simulink model "CM012A_FordT3McuCfg"  (R2013b)
settings: Solver=FixedStepDiscrete  SolverMode=SingleTasking  StartTime=0.0  StopTime=2  FixedStep=0.00005  RelTol=1e-3
values from neighbouring files (symbols this model uses):
  BATTVLTGSCAGFAC_ULS_F32 = DataDict.Constant    [CM012A_FordT3McuCfg_DataDict.m]
  BATTVLTGSWD1SCAGFAC_ULS_F32 = DataDict.Constant    [CM012A_FordT3McuCfg_DataDict.m]
  CHRGPMPDIAGSCAGFAC_ULS_F32 = DataDict.Constant    [CM012A_FordT3McuCfg_DataDict.m]
  MOTAG2MEAS_ECU1OFFS_MOTREV_F32 = DataDict.Constant    [CM012A_FordT3McuCfg_DataDict.m]
  MOTAG2MEAS_ECU2OFFS_MOTREV_F32 = DataDict.Constant    [CM012A_FordT3McuCfg_DataDict.m]
  PWRDISCNCTSWTDIAGSCAGFAC_ULS_F32 = DataDict.Constant    [CM012A_FordT3McuCfg_DataDict.m]
undefined symbols (not defined in the file or in its folder): HwAgSnsrTyp1, sigbuilder_block
libraries: CM012A_FordT3McuCfg_ModelLibrary x114, simulink x37, NxtrLim x34
(part 1 of 4)
settings Model: Creator=nz3zln  LastModifiedBy=NZ4630
settings SolverCC: AutoInsertRateTranBlk=on  InsertRTBMode=Always
settings DataIOCC: LimitDataPoints=off  SaveFormat=Structure  ReturnWorkspaceOutputs=on
settings OptimizationCC: BlockReduction=off  InlineParams=on  ZeroExternalMemoryAtStartup=off  ZeroInternalMemoryAtStartup=off  OptimizeModelRefInitCode=on  LifeSpan=1
settings DebuggingCC: SignalInfNanChecking=error  SignalRangeChecking=warning  UnderspecifiedInitializationDetection=Simplified  SolverPrmCheckMsg=error  InheritedTsInSrcMsg=error  DiscreteInheritContinuousMsg=error  MultiTaskRateTransMsg=warning  SingleTaskRateTransMsg=error  TasksWithSamePriorityMsg=error  SigSpecEnsureSampleTimeMsg=error  CheckMatrixSingularityMsg=error  ParameterUnderflowMsg=error  ParameterPrecisionLossMsg=none  ParameterTunabilityLossMsg=error  FixptConstUnderflowMsg=warning  FixptConstOverflowMsg=warning  VectorMatrixConversionMsg=error  SignalLabelMismatchMsg=error  UnconnectedInputMsg=error  UnconnectedOutputMsg=error  UnconnectedLineMsg=error  SFcnCompatibilityMsg=error  UniqueDataStoreMsg=warning  BusObjectLabelMismatch=error  RootOutportRequireBusObject=error  AssertControl=DisableAll  ModelReferenceIOMsg=error  ModelReferenceVersionMismatchMessage=warning  ModelReferenceIOMismatchMessage=error  ModelReferenceCSMismatchMessage=warning  ModelReferenceDataLoggingMessage=error  StateNameClashWarn=warning  StrictBusMsg=ErrorOnBusTreatedAsVector  NonBusSignalsTreatedAsBus=error  SFUnexpectedBacktrackingDiag=error  SFInvalidInputDataAccessInChartInitDiag=error  SFNoUnconditionalDefaultTransitionDiag=error  SFTransitionOutsideNaturalParentDiag=error  SFUnconditionalTransitionShadowingDiag=error  SFUndirectedBroadcastEventsDiag=error
settings ModelReferenceCC: ModelReferenceNumInstancesAllowed=Single
settings RTWCC: SystemTargetFile=autosar.tlc  GenCodeOnly=on  TemplateMakefile=ert_default_tmf  Description=AUTOSAR  GenerateReport=on  ProcessScript=autosar_make_rtw_hook  LaunchReport=on
settings CodeAppCC: GenerateComments=off  IgnoreCustomStorageClasses=off  CustomSymbolStrType=$N$R$M  CustomSymbolStrBlkIO=$N$M  SimulinkBlockComments=off
settings STFCustomTargetCC: ParMdlRefBuildCompliant=on  CompOptLevelCompliant=on  IncludeMdlTerminateFcn=off  CombineOutputUpdateFcns=on  SuppressErrorStatus=on  ERTFirstTimeCompliant=on  ERTCustomFileBanners=on  SupportNonFinite=off  SupportComplex=off  SupportContinuousTime=off  SupportNonInlinedSFcns=off  MATLABClassNameForMDSCustomization=Simulink.SoftwareTarget.ERTCustomization  AutosarCompliant=on  GRTInterface=off  SystemTargetFile=autosar.tlc
settings ERTTargetCC: CodeReplacementLibrary=ANSI_C  ConcurrentExecutionCompliant=off  IncludeMdlTerminateFcn=off  SuppressErrorStatus=on  SupportNonFinite=off  SupportComplex=off  ModelStepFunctionPrototypeControlCompliant=off  CPPClassGenCompliant=off  AutosarCompliant=on  InlinedParameterPlacement=NonHierarchical  ERTCustomFileTemplate=example_file_process.tlc  EnableUserReplacementTypes=on

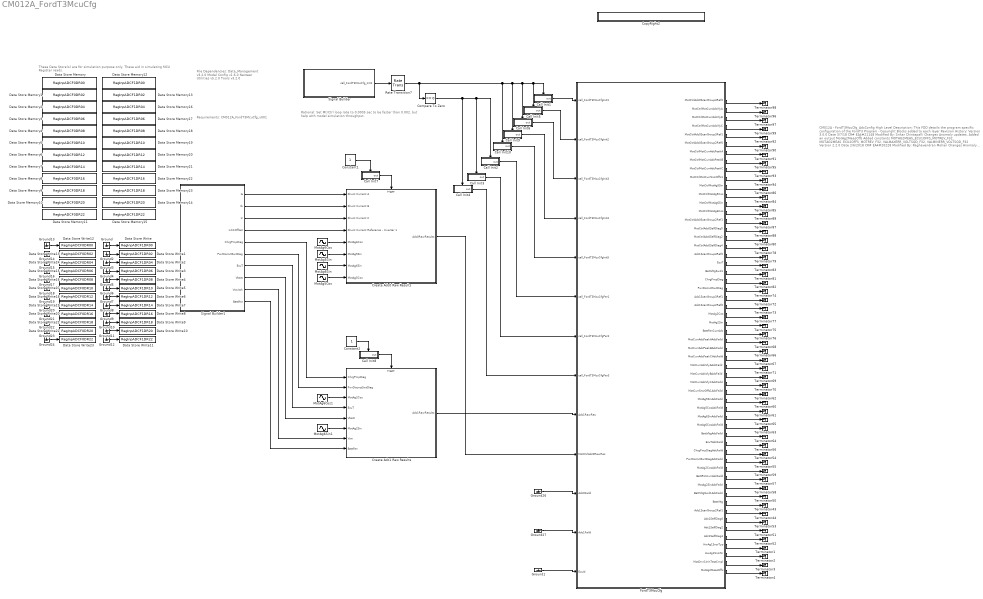
== system CM012A_FordT3McuCfg ==
  note: These Data Store(s) are for simulation purpose only, These aid in simulating MCU
      | Register reads.
  note: File Dependencies:
      |
      | Data_Management v3.2.0
      | Model Config v1.6.0
      | Nexteer Utilities v5.2.0
      | Tools v3.2.0
  note: CM012A - FordT3McuCfg_AdcConfig
      |
      | High Level Description:
      | This FDD details the program specific configuration of the FordT3 Program
      |  - Copyright Blocks added to each layer
      |
      | Revision History:
      |
      | Version		3.0.0
      | Date 		3/7/18
      | CR#		EA4#21148
      | Modified By: 	Srikar Chintapalli
      | Changes		Anomaly updates,
      |                       Added an output MotAg2MeasOffs
      | 			Added constants MOTAG2MEAS_ECU1OFFS_MOTREV_F32,
      |                       MOTAG2MEAS_ECU2OFFS_MOTREV_F32,
      |                       VALMAXERR_VOLTSQD_F32, VALMINERR_VOLTSQD_F32
      |
      |
      | Version		2.2.0
      | Date 		2/6/2018
      | CR#		EA4#20228
      | Modified By: 	Raghavendran Mohan
      | Changes		Anomaly updates,
      | 			Updated (.m) DataDict file,
      | 			ECUTMEAS_FILTAU_HZ_F32 = 2;
      | 			ECUTMEAS_RNGDIAGCMAX_DEGCGRD_F32 = 125;
      | 			ECUTMEAS_RNGDIAGCMIN_DEGCGRD_F32 = -40;
      |
      | 			Port Config spreadsheet
      | 			Updated All SENT peripherals to have high port drive strength.
      | 			Updated Handwheel torque signal names and FDD names.
      |
      | 			AdcConfig spreadsheet, FordT3McuCfgAndUse.vsd
      | 			Swapped the virtual channel naming for Peak and Valley motor current reads.
      |
      | 			SensorAbstraction spreadsheet,
      | 			Updated Motor angle and Handwheel torque component list.
      |
      | Version		2.1.0
      | Date 		11/30/2017
      | CR#		EA4#17822
      | Modified By: 	Raghavendran Mohan
      | Changes		- Modified EngVal for ECUTMEAS_ECUTX_VOLT_U3P13 and
      | 		         ECUTMEAS_ECUTY_DEGCGRD_S8P7 in the DataDict file.
      | 			- Modified PIBC for ECUID1.
      | 			- Renamed HwTrq 1 and HwTrq8 in the PortConfig File.
      | 			- Removed Writes to MSR_LM2 register to avoid guard errors.
      | 				(powerdownmoderegister).
      |
      | Version		2.0.0
      | Date 		9/5/2017
      | CR#		EA4#12623
      | Modified By: 	Raghavendran Mohan
      | Changes		- Added MotDrvr1IninTestCmpl as an output.
      | 			- Updated Call locations.
      | 			- Updated Inverter Count ELECGLBPRM_IVTRCNT_CNT_U08
      | 			   to have value of 1 in (.m) DataDict file.
      | 			- Updated ECU ID Pin2. (PortConfig Excel).
      | 			- Updated GateDrive Signal names to GateDrive0 in PortConfig.
      | 			- Updated power supply SPI channel select as alternate output in PortConfig.
      | 			- Updated HwTrq components to be corresponding alternate outputs in PortConfig.
      | 			- Updated Hw Torque and Hw Angle Sensor Ntc information in DataDict.
      |
      | Version		1.0.0
      | Date 		7/24/2017
      | CR#		EA4#12623
      | Modified By: 	Raghavendran Mohan
      | Changes		Initial Release
  note: Requirements:
      |
      | CM012A_FordT3McuCfg_v001
  note: Rational:
      |
      | Set MtrCtrl loop rate to 0.0005 sec to be
      | faster than 0.002, but help with model simulation
      | throughput.
  Call Init1 : Subsystem  TreatAsAtomicUnit=on
  Call Init10 : Subsystem  TreatAsAtomicUnit=on
  Call Init2 : Subsystem  TreatAsAtomicUnit=on
  Call Init3 : Subsystem  TreatAsAtomicUnit=on
  Call Init4 : Subsystem  TreatAsAtomicUnit=on
  Call Init5 : Subsystem  TreatAsAtomicUnit=on
  Call Init6 : Subsystem  TreatAsAtomicUnit=on
  Call Init7 : Subsystem  TreatAsAtomicUnit=on
  Call Init8 : Subsystem  TreatAsAtomicUnit=on
  Call Init9 : Subsystem  TreatAsAtomicUnit=on
  Compare To Zero : simulink/Logic and Bit Operations/Compare To Zero  relop===  OutDataTypeStr=uint8
  Constant1 : Constant  OutDataTypeStr=int8
  Constant2 : Constant  OutDataTypeStr=int8
  CopyRight2 : Subsystem  Description=|  mask(Copyright Information){none=on}
      | Copyright info block.                                               
      |                                                                     
      | Place copyright information at the top of every subsystem in design.
      mask prompts: none "No parameters"
      mask help: Place copyright information at the top of every subsystem in design.
      mask Display:
      | NxtrConf = 'Nexteer Confidential';
      | 
      | sys = bdroot; %handle for the current model ("system")
      | first = get_param(sys,'Created');
      | first = first(end-3:end);  %year is last four digits
      | 
      | last = get_param(sys,'LastModifiedDate');
      | if isempty(last)
      |     last = datestr(now,'yyyy');
      | else
      |     last = last(end-3:end);
      | end
      | 
      | if strcmp(first,last)
      |     fprintf('%s -- Copyright %s Nexteer',NxtrConf,first)
      | else
      |     fprintf('%s -- %s%s- %s Nexteer',NxtrConf,char(169),first,last)
      | end
  Create Adc0 Raw Results : Subsystem
  Create Adc1 Raw Results : Subsystem
  Data Store Memory : DataStoreMemory  DataStoreName=RegInpADCF0DR00  OutDataTypeStr=uint32
  Data Store Memory1 : DataStoreMemory  DataStoreName=RegInpADCF0DR02  OutDataTypeStr=uint32
  Data Store Memory10 : DataStoreMemory  DataStoreName=RegInpADCF0DR20  OutDataTypeStr=uint32
  Data Store Memory11 : DataStoreMemory  DataStoreName=RegInpADCF0DR22  OutDataTypeStr=uint32
  Data Store Memory12 : DataStoreMemory  DataStoreName=RegInpADCF1DR00  OutDataTypeStr=uint32
  Data Store Memory13 : DataStoreMemory  DataStoreName=RegInpADCF1DR02  OutDataTypeStr=uint32
  Data Store Memory14 : DataStoreMemory  DataStoreName=RegInpADCF1DR20  OutDataTypeStr=uint32
  Data Store Memory15 : DataStoreMemory  DataStoreName=RegInpADCF1DR22  OutDataTypeStr=uint32
  Data Store Memory16 : DataStoreMemory  DataStoreName=RegInpADCF1DR04  OutDataTypeStr=uint32
  Data Store Memory17 : DataStoreMemory  DataStoreName=RegInpADCF1DR06  OutDataTypeStr=uint32
  Data Store Memory18 : DataStoreMemory  DataStoreName=RegInpADCF1DR08  OutDataTypeStr=uint32
  Data Store Memory19 : DataStoreMemory  DataStoreName=RegInpADCF1DR10  OutDataTypeStr=uint32
  Data Store Memory2 : DataStoreMemory  DataStoreName=RegInpADCF0DR04  OutDataTypeStr=uint32
  Data Store Memory20 : DataStoreMemory  DataStoreName=RegInpADCF1DR12  OutDataTypeStr=uint32
  Data Store Memory21 : DataStoreMemory  DataStoreName=RegInpADCF1DR14  OutDataTypeStr=uint32
  Data Store Memory22 : DataStoreMemory  DataStoreName=RegInpADCF1DR16  OutDataTypeStr=uint32
  Data Store Memory23 : DataStoreMemory  DataStoreName=RegInpADCF1DR18  OutDataTypeStr=uint32
  Data Store Memory3 : DataStoreMemory  DataStoreName=RegInpADCF0DR06  OutDataTypeStr=uint32
  Data Store Memory4 : DataStoreMemory  DataStoreName=RegInpADCF0DR08  OutDataTypeStr=uint32
  Data Store Memory5 : DataStoreMemory  DataStoreName=RegInpADCF0DR10  OutDataTypeStr=uint32
  Data Store Memory6 : DataStoreMemory  DataStoreName=RegInpADCF0DR12  OutDataTypeStr=uint32
  Data Store Memory7 : DataStoreMemory  DataStoreName=RegInpADCF0DR14  OutDataTypeStr=uint32
  Data Store Memory8 : DataStoreMemory  DataStoreName=RegInpADCF0DR16  OutDataTypeStr=uint32
  Data Store Memory9 : DataStoreMemory  DataStoreName=RegInpADCF0DR18  OutDataTypeStr=uint32
  Data Store Write : DataStoreWrite  DataStoreName=RegInpADCF1DR00
  Data Store Write1 : DataStoreWrite  DataStoreName=RegInpADCF1DR02
  Data Store Write10 : DataStoreWrite  DataStoreName=RegInpADCF1DR20
  Data Store Write11 : DataStoreWrite  DataStoreName=RegInpADCF1DR22
  Data Store Write12 : DataStoreWrite  DataStoreName=RegInpADCF0DR00
  Data Store Write13 : DataStoreWrite  DataStoreName=RegInpADCF0DR02
  Data Store Write14 : DataStoreWrite  DataStoreName=RegInpADCF0DR04
  Data Store Write15 : DataStoreWrite  DataStoreName=RegInpADCF0DR06
  Data Store Write16 : DataStoreWrite  DataStoreName=RegInpADCF0DR08
  Data Store Write17 : DataStoreWrite  DataStoreName=RegInpADCF0DR10
  Data Store Write18 : DataStoreWrite  DataStoreName=RegInpADCF0DR12
  Data Store Write19 : DataStoreWrite  DataStoreName=RegInpADCF0DR14
  Data Store Write2 : DataStoreWrite  DataStoreName=RegInpADCF1DR04
  Data Store Write20 : DataStoreWrite  DataStoreName=RegInpADCF0DR16
  Data Store Write21 : DataStoreWrite  DataStoreName=RegInpADCF0DR18
  Data Store Write22 : DataStoreWrite  DataStoreName=RegInpADCF0DR20
  Data Store Write23 : DataStoreWrite  DataStoreName=RegInpADCF0DR22
  Data Store Write3 : DataStoreWrite  DataStoreName=RegInpADCF1DR06
  Data Store Write4 : DataStoreWrite  DataStoreName=RegInpADCF1DR08
  Data Store Write5 : DataStoreWrite  DataStoreName=RegInpADCF1DR10
  Data Store Write6 : DataStoreWrite  DataStoreName=RegInpADCF1DR12
  Data Store Write7 : DataStoreWrite  DataStoreName=RegInpADCF1DR14
  Data Store Write8 : DataStoreWrite  DataStoreName=RegInpADCF1DR16
  Data Store Write9 : DataStoreWrite  DataStoreName=RegInpADCF1DR18
  FordT3McuCfg : Subsystem
  Ground{,1..24,26..27} (27 alike) : Ground
  MotAg5Cos : Sin  Bias=1  Frequency=500  Phase=pi/2  SampleTime=0
  MotAg5Sin : Sin  Bias=1  Frequency=500  SampleTime=0
  MotAg6Cos : Sin  Bias=1  Frequency=1000  Phase=pi/2  SampleTime=0
  MotAg6Cos1 : Sin  Bias=1  Frequency=750  Phase=pi/2  SampleTime=0
  MotAg6Sin : Sin  Bias=1  Frequency=1000  SampleTime=0
  MotAg6Sin1 : Sin  Bias=1  Frequency=750  SampleTime=0
  Rate Transition7 : RateTransition
  Signal Builder : Subsystem  Tag=STV Subsys  RequirementInfo={} %GIDa_2822100e_29fa_4197_9ccc_01864625f252  LoadFcn=sigbuilder_block('load');  StartFcn=sigbuilder_block('start');  StopFcn=sigbuilder_block('stop');  ClipboardFcn=sigbuilder_block('clipboard');  mask(Sigbuilder block){}
      mask help: Simulink:masks:SigbuilderBlock_MD
      mask init:
      | if ~strcmp(get_param(bdroot(gcbh),'SimulationStatus'),'stopped') tuvar = sigbuilder_block('maskInit'); end
      settings: CopyFcn=sigbuilder_block('copy');  DeleteFcn=sigbuilder_block('delete');  ModelCloseFcn=sigbuilder_block('modelClose');  PreSaveFcn=sigbuilder_block('preSave');  PauseFcn=sigbuilder_block('pause');  ContinueFcn=sigbuilder_block('continue');  NameChangeFcn=sigbuilder_block('namechange');  OpenFcn=sigbuilder_block('open',[5.58621 7.44828 1178.69 604.552 ]);  CloseFcn=sigbuilder_block('close');
      mask Display: plot(0, 0, 100, 100,[2, 2, 32, 32, 2], [68, 8, 8, 68, 68],[32, 2], [38, 38], [32, 19, 2],[53, 60, 44], [32, 17, 17, 2],[16, 16, 31, 31]);txt = getActiveGroup(gcbh);text(2, 100, txt,'verticalAlignment', 'top');
  Signal Builder1 : Subsystem  Tag=STV Subsys  LoadFcn=sigbuilder_block('load');  StartFcn=sigbuilder_block('start');  StopFcn=sigbuilder_block('stop');  ClipboardFcn=sigbuilder_block('clipboard');  mask(Sigbuilder block){}
      mask help: Simulink:masks:SigbuilderBlock_MD
      mask init:
      | if ~strcmp(get_param(bdroot(gcbh),'SimulationStatus'),'stopped') tuvar = sigbuilder_block('maskInit'); end
      settings: CopyFcn=sigbuilder_block('copy');  DeleteFcn=sigbuilder_block('delete');  ModelCloseFcn=sigbuilder_block('modelClose');  PreSaveFcn=sigbuilder_block('preSave');  PauseFcn=sigbuilder_block('pause');  ContinueFcn=sigbuilder_block('continue');  NameChangeFcn=sigbuilder_block('namechange');  OpenFcn=sigbuilder_block('open',[0 29.7931 1191.72 587.172 ]);  CloseFcn=sigbuilder_block('close');
      mask Display: plot(0, 0, 100, 100,[2, 2, 32, 32, 2], [68, 8, 8, 68, 68],[32, 2], [38, 38], [32, 19, 2],[53, 60, 44], [32, 17, 17, 2],[16, 16, 31, 31]);txt = getActiveGroup(gcbh);text(2, 100, txt,'verticalAlignment', 'top');
  Terminator{1..4,43..44,50..99} (56 alike) : Terminator
  wires:
  Signal Builder/1(call_FordT3McuCfg_Init1) -> Rate Transition7/1
  Constant1/1 -> Call Init7/Enable
  Call Init7/1(out) -> Create Adc0 Raw Results/Trigger
  Constant2/1 -> Call Init8/Enable
  Call Init8/1(out) -> Create Adc1 Raw Results/Trigger
  FordT3McuCfg/47(BattVltgSwd1AdcFaild) -> Terminator50/1
  FordT3McuCfg/48(BattVltg) -> Terminator43/1
  FordT3McuCfg/49(Adc1ScanGroup2Ref1) -> Terminator44/1
  FordT3McuCfg/50(Adc1SelfDiag0) -> Terminator53/1
  FordT3McuCfg/51(Adc1SelfDiag2) -> Terminator51/1
  FordT3McuCfg/52(Adc1SelfDiag4) -> Terminator52/1
  FordT3McuCfg/41(EcuTAdcFaild) -> Terminator56/1
  FordT3McuCfg/42(ChrgPmpDiagAdcFaild) -> Terminator54/1
  FordT3McuCfg/43(PwrDiscnctSwtDiagAdcFaild) -> Terminator55/1
  FordT3McuCfg/44(MotAg2CosAdcFaild) -> Terminator59/1
  FordT3McuCfg/45(BattRtnCurrAdcFaild) -> Terminator57/1
  FordT3McuCfg/46(MotAg2SinAdcFaild) -> Terminator58/1
  FordT3McuCfg/35(MotCurrSnsrOffs1AdcFaild) -> Terminator62/1
  FordT3McuCfg/36(MotAg5SinAdcFaild) -> Terminator60/1
  FordT3McuCfg/37(MotAg5CosAdcFaild) -> Terminator61/1
  FordT3McuCfg/38(MotAg6SinAdcFaild) -> Terminator65/1
  FordT3McuCfg/39(MotAg6CosAdcFaild) -> Terminator63/1
  FordT3McuCfg/40(BattVltgAdcFaild) -> Terminator64/1
  FordT3McuCfg/29(MotCurrAdcPeakAAdcFaild) -> Terminator68/1
  FordT3McuCfg/30(MotCurrAdcPeakBAdcFaild) -> Terminator66/1
  FordT3McuCfg/31(MotCurrAdcPeakCAdcFaild) -> Terminator67/1
  FordT3McuCfg/32(MotCurrAdcVlyAAdcFaild) -> Terminator71/1
  FordT3McuCfg/33(MotCurrAdcVlyBAdcFaild) -> Terminator69/1
  FordT3McuCfg/34(MotCurrAdcVlyCAdcFaild) -> Terminator70/1
  FordT3McuCfg/23(PwrDiscnctSwtDiag) -> Terminator74/1
  FordT3McuCfg/24(Adc1ScanGroup3Ref1) -> Terminator72/1
  FordT3McuCfg/25(Adc1ScanGroup2Ref0) -> Terminator73/1
  FordT3McuCfg/26(MotAg2Cos) -> Terminator77/1
  FordT3McuCfg/27(MotAg2Sin) -> Terminator75/1
  FordT3McuCfg/28(BattRtnCurrAdc) -> Terminator76/1
  FordT3McuCfg/17(MotCtrlAdc0SelfDiag2) -> Terminator80/1
  FordT3McuCfg/18(MotCtrlAdc0SelfDiag4) -> Terminator78/1
  FordT3McuCfg/19(Adc1ScanGroup3Ref0) -> Terminator79/1
  FordT3McuCfg/20(EcuT) -> Terminator83/1
  FordT3McuCfg/21(BattVltgSwd1) -> Terminator81/1
  FordT3McuCfg/22(ChrgPmpDiag) -> Terminator82/1
  FordT3McuCfg/11(MotCtrlMotAg5Sin) -> Terminator86/1
  FordT3McuCfg/12(MotCtrlMotAg5Cos) -> Terminator84/1
  FordT3McuCfg/13(MotCtrlMotAg6Sin) -> Terminator85/1
  FordT3McuCfg/14(MotCtrlMotAg6Cos) -> Terminator89/1
  FordT3McuCfg/15(MotCtrlAdc0ScanGroup2Ref1) -> Terminator87/1
  FordT3McuCfg/16(MotCtrlAdc0SelfDiag0) -> Terminator88/1
  FordT3McuCfg/5(MotCtrlAdc0ScanGroup3Ref1) -> Terminator92/1
  FordT3McuCfg/6(MotCtrlAdc0ScanGroup2Ref0) -> Terminator90/1
  FordT3McuCfg/7(MotCtrlMotCurrAdcPeakA) -> Terminator91/1
  FordT3McuCfg/8(MotCtrlMotCurrAdcPeakB) -> Terminator95/1
  FordT3McuCfg/9(MotCtrlMotCurrAdcPeakC) -> Terminator93/1
  FordT3McuCfg/10(MotCtrlMotCurrSnsrOffs1) -> Terminator94/1
  FordT3McuCfg/1(MotCtrlAdc0ScanGroup3Ref0) -> Terminator98/1
  FordT3McuCfg/2(MotCtrlMotCurrAdcVlyA) -> Terminator96/1
  FordT3McuCfg/3(MotCtrlMotCurrAdcVlyB) -> Terminator97/1
  FordT3McuCfg/4(MotCtrlMotCurrAdcVlyC) -> Terminator99/1
  Signal Builder1/1(Ia) -> Create Adc0 Raw Results/1(Shunt Current A)
  Signal Builder1/2(Ib) -> Create Adc0 Raw Results/2(Shunt Current B)
  Signal Builder1/3(Ic) -> Create Adc0 Raw Results/3(Shunt Current C)
  Signal Builder1/4(Ivtr1Offset) -> Create Adc0 Raw Results/4(Shunt Current Reference - Inverter 1)
  MotAg5Cos/1 -> Create Adc0 Raw Results/8(MotAg5Cos)
  MotAg6Cos/1 -> Create Adc0 Raw Results/5(MotAg6Cos)
  MotAg6Sin/1 -> Create Adc0 Raw Results/7(MotAg6Sin)
  MotAg6Cos1/1 -> Create Adc1 Raw Results/3(MotAg2Cos)
  MotAg6Sin1/1 -> Create Adc1 Raw Results/6(MotAg2Sin)
  Signal Builder1/5(ChrgPmpDiag) -> Create Adc1 Raw Results/1(ChrgPmpDiag)
  Signal Builder1/6(PwrDiscnctSwtDiag) -> Create Adc1 Raw Results/2(PwrDiscnctSwtDiag)
  Signal Builder1/8(Vbatt) -> Create Adc1 Raw Results/5(Vbatt)
  Signal Builder1/7(EcuT) -> Create Adc1 Raw Results/4(EcuT)
  Signal Builder1/9(Vswitch) -> Create Adc1 Raw Results/7(Vsw)
  Signal Builder1/10(BattRtn) -> Create Adc1 Raw Results/8(BattRtn)
  Compare To Zero/1 -> Call Init4/Enable, Call Init3/Enable, Call Init2/Enable
  FordT3McuCfg/53(HwAg1SnsrTyp) -> Terminator1/1
  FordT3McuCfg/54(HwAg1SnsrNr) -> Terminator2/1
  MotAg5Sin/1 -> Create Adc0 Raw Results/6(MotAg5Sin)
  Ground/1 -> Data Store Write/1
  Ground2/1 -> Data Store Write1/1
  Ground3/1 -> Data Store Write2/1
  Ground4/1 -> Data Store Write3/1
  Ground5/1 -> Data Store Write4/1
  Ground6/1 -> Data Store Write5/1
  Ground7/1 -> Data Store Write6/1
  Ground8/1 -> Data Store Write7/1
  Ground9/1 -> Data Store Write8/1
  Ground10/1 -> Data Store Write9/1
  Ground11/1 -> Data Store Write10/1
  Ground12/1 -> Data Store Write11/1
  Ground13/1 -> Data Store Write12/1
  Ground14/1 -> Data Store Write13/1
  Ground15/1 -> Data Store Write14/1
  Ground16/1 -> Data Store Write15/1
  Ground17/1 -> Data Store Write16/1
  Ground18/1 -> Data Store Write17/1
  Ground19/1 -> Data Store Write18/1
  Ground20/1 -> Data Store Write19/1
  Ground21/1 -> Data Store Write20/1
  Ground22/1 -> Data Store Write21/1
  Ground23/1 -> Data Store Write22/1
  Ground24/1 -> Data Store Write23/1
  FordT3McuCfg/55(MotDrvr1IninTestCmpl) -> Terminator3/1
  Call Init1/1(out) -> FordT3McuCfg/1(call_FordT3McuCfgInit1)
  Call Init5/1(out) -> FordT3McuCfg/2(call_FordT3McuCfgInit2)
  Call Init6/1(out) -> FordT3McuCfg/3(call_FordT3McuCfgInit3)
  Call Init9/1(out) -> FordT3McuCfg/4(call_FordT3McuCfgInit4)
  Rate Transition7/1 -> Compare To Zero/1, Call Init1/Enable, Call Init5/Enable, Call Init6/Enable, Call Init9/Enable, Call Init10/Enable
  Call Init10/1(out) -> FordT3McuCfg/5(call_FordT3McuCfgInit5)
  Ground27/1 -> FordT3McuCfg/12(Adc1Faild)
  Ground26/1 -> FordT3McuCfg/11(Adc0Faild)
  Ground1/1 -> FordT3McuCfg/13(EcuId)
  Call Init2/1(out) -> FordT3McuCfg/6(call_FordT3McuCfgPer1)
  Call Init3/1(out) -> FordT3McuCfg/7(call_FordT3McuCfgPer2)
  Call Init4/1(out) -> FordT3McuCfg/8(call_FordT3McuCfgPer3)
  Create Adc1 Raw Results/1(Adc1RawResults) -> FordT3McuCfg/9(Adc1RawRes)
  Create Adc0 Raw Results/1(Adc0RawResults) -> FordT3McuCfg/10(MotCtrlAdc0RawRes)
  FordT3McuCfg/56(MotAg2MeasOffs) -> Terminator4/1

== system CM012A_FordT3McuCfg/Call Init1 ==
  Enable : EnablePort
  Function Call Trigger : simulink/Ports & Subsystems/Function-Call Generator  RequirementInfo={} %GIDa_ff755a2e_49d1_45f7_8591_3ce0ef475338  sample_time=0.002  numberOfIterations=1
  out : Outport
  wires:
  Function Call Trigger/1 -> out/1

== system CM012A_FordT3McuCfg/Call Init10 ==
  Enable : EnablePort
  Function Call Trigger : simulink/Ports & Subsystems/Function-Call Generator  RequirementInfo={} %GIDa_64d9d107_69c6_4fb8_b290_e9fb46496850  sample_time=0.002  numberOfIterations=1
  out : Outport
  wires:
  Function Call Trigger/1 -> out/1

== system CM012A_FordT3McuCfg/Call Init2 ==
  Enable : EnablePort
  Function Call Trigger : simulink/Ports & Subsystems/Function-Call Generator  RequirementInfo={} %GIDa_ba5be832_aeac_40ae_ae53_3fd25198366e  sample_time=0.00005  numberOfIterations=1
  out : Outport
  wires:
  Function Call Trigger/1 -> out/1

== system CM012A_FordT3McuCfg/Call Init3 ==
  Enable : EnablePort
  Function Call Trigger : simulink/Ports & Subsystems/Function-Call Generator  RequirementInfo={} %GIDa_bf682727_f4b1_4f52_ae72_c6f6d8d412d7  sample_time=0.002  numberOfIterations=1
  out : Outport
  wires:
  Function Call Trigger/1 -> out/1

== system CM012A_FordT3McuCfg/Call Init4 ==
  Enable : EnablePort
  Function Call Trigger : simulink/Ports & Subsystems/Function-Call Generator  RequirementInfo={} %GIDa_39162fcb_260a_4191_9640_bf2fa4fe87e2  sample_time=0.002  numberOfIterations=1
  out : Outport
  wires:
  Function Call Trigger/1 -> out/1

== system CM012A_FordT3McuCfg/Call Init5 ==
  Enable : EnablePort
  Function Call Trigger : simulink/Ports & Subsystems/Function-Call Generator  RequirementInfo={} %GIDa_52b82f2d_d21e_4ccf_9b87_2b660c433421  sample_time=0.002  numberOfIterations=1
  out : Outport
  wires:
  Function Call Trigger/1 -> out/1

== system CM012A_FordT3McuCfg/Call Init6 ==
  Enable : EnablePort
  Function Call Trigger : simulink/Ports & Subsystems/Function-Call Generator  RequirementInfo={} %GIDa_40b20fc1_ef82_4ce8_9bb2_77ecb7477d85  sample_time=0.00005  numberOfIterations=1
  out : Outport
  wires:
  Function Call Trigger/1 -> out/1

== system CM012A_FordT3McuCfg/Call Init7 ==
  Enable : EnablePort
  Function Call Trigger : simulink/Ports & Subsystems/Function-Call Generator  RequirementInfo={} %GIDa_6dd05ab1_f91b_4d7a_a0ec_1170d213fa7b  sample_time=0.0005  numberOfIterations=1
  out : Outport
  wires:
  Function Call Trigger/1 -> out/1

== system CM012A_FordT3McuCfg/Call Init8 ==
  Enable : EnablePort
  Function Call Trigger : simulink/Ports & Subsystems/Function-Call Generator  RequirementInfo={} %GIDa_1bbba36e_83d5_4174_9ee1_08e29d90f8ad  sample_time=0.002  numberOfIterations=1
  out : Outport
  wires:
  Function Call Trigger/1 -> out/1

== system CM012A_FordT3McuCfg/Call Init9 ==
  Enable : EnablePort
  Function Call Trigger : simulink/Ports & Subsystems/Function-Call Generator  RequirementInfo={} %GIDa_802b6c3d_d439_41e3_9021_697c35b24e20  sample_time=0.002  numberOfIterations=1
  out : Outport
  wires:
  Function Call Trigger/1 -> out/1

== system CM012A_FordT3McuCfg/CopyRight2 ==

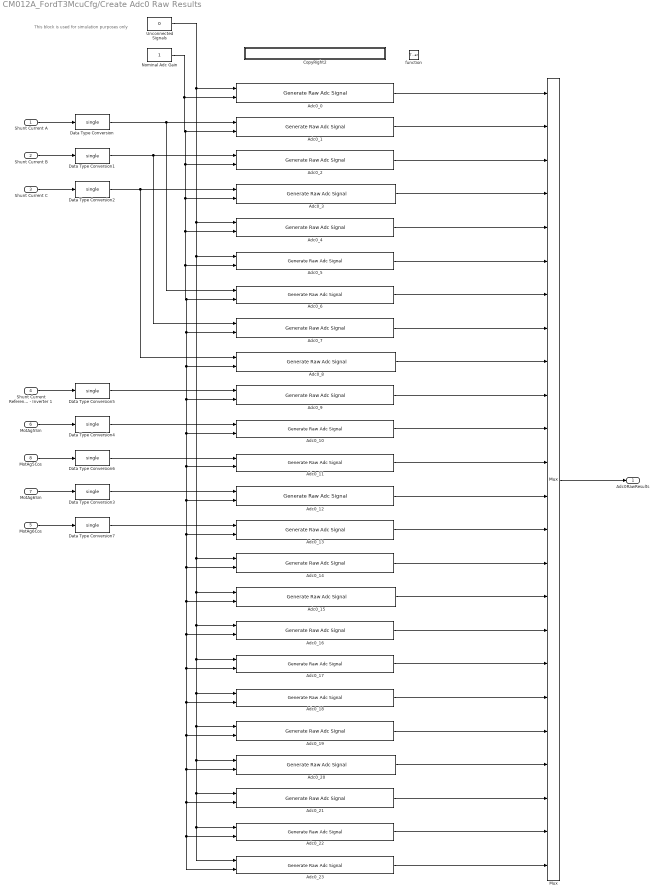
== system CM012A_FordT3McuCfg/Create Adc0 Raw Results ==
  note: This block is used for simulation purposes only
  Shunt Current A : Inport  RequirementInfo={} %GIDa_668e5a0c_60cb_44fa_a0aa_319a7fa0b265
  Shunt Current B : Inport  RequirementInfo={} %GIDa_16ae5539_98f1_4c07_920b_74e858da5360  Port=2
  Shunt Current C : Inport  RequirementInfo={} %GIDa_2e65608c_dfbe_4411_b06e_4614975fb2b8  Port=3
  Shunt Current Reference - Inverter 1 : Inport  RequirementInfo={} %GIDa_cdc72450_9145_46a4_94e4_915d846ab52f  Port=4
  MotAg6Cos : Inport  RequirementInfo={} %GIDa_2b4fc733_1ee0_4c0f_9d62_aa17fffd2420  Port=5
  MotAg5Sin : Inport  RequirementInfo={} %GIDa_cfee6a52_2a0a_4bc7_8546_14dd79a467e4  Port=6
  MotAg6Sin : Inport  RequirementInfo={} %GIDa_cf4c08a2_d259_4630_af2a_9be94b72bff3  Port=7
  MotAg5Cos : Inport  RequirementInfo={} %GIDa_b3cf61d5_a897_4d0a_a815_ae22db780a99  Port=8
  function : TriggerPort  TriggerType=function-call
  Adc0_{0..23} (24 alike) : CM012A_FordT3McuCfg_ModelLibrary/Generate Raw Adc Signal
  CopyRight2 : Subsystem  Description=|  mask(Copyright Information){none=on}
      | Copyright info block.                                               
      |                                                                     
      | Place copyright information at the top of every subsystem in design.
      mask prompts: none "No parameters"
      mask help: Place copyright information at the top of every subsystem in design.
      mask Display:
      | NxtrConf = 'Nexteer Confidential';
      | 
      | sys = bdroot; %handle for the current model ("system")
      | first = get_param(sys,'Created');
      | first = first(end-3:end);  %year is last four digits
      | 
      | last = get_param(sys,'LastModifiedDate');
      | if isempty(last)
      |     last = datestr(now,'yyyy');
      | else
      |     last = last(end-3:end);
      | end
      | 
      | if strcmp(first,last)
      |     fprintf('%s -- Copyright %s Nexteer',NxtrConf,first)
      | else
      |     fprintf('%s -- %s%s- %s Nexteer',NxtrConf,char(169),first,last)
      | end
  Data Type Conversion{,1..7} (8 alike) : DataTypeConversion  OutDataTypeStr=single
  Mux : Mux  Inputs=24
  Nominal Adc Gain : Constant  OutDataTypeStr=single
  Unconnected Signals : Constant  Value=0  OutDataTypeStr=single
  Adc0RawResults : Outport
  wires:
  Mux/1 -> Adc0RawResults/1
  Adc0_0/1 -> Mux/1
  Adc0_1/1 -> Mux/2
  Adc0_2/1 -> Mux/3
  Adc0_3/1 -> Mux/4
  Adc0_4/1 -> Mux/5
  Adc0_5/1 -> Mux/6
  Adc0_6/1 -> Mux/7
  Adc0_7/1 -> Mux/8
  Adc0_8/1 -> Mux/9
  Adc0_9/1 -> Mux/10
  Adc0_10/1 -> Mux/11
  Adc0_11/1 -> Mux/12
  Adc0_12/1 -> Mux/13
  Adc0_13/1 -> Mux/14
  Adc0_14/1 -> Mux/15
  Adc0_15/1 -> Mux/16
  Adc0_16/1 -> Mux/17
  Adc0_17/1 -> Mux/18
  Adc0_18/1 -> Mux/19
  Adc0_19/1 -> Mux/20
  Adc0_20/1 -> Mux/21
  Adc0_21/1 -> Mux/22
  Adc0_22/1 -> Mux/23
  Adc0_23/1 -> Mux/24
  Unconnected Signals/1 -> Adc0_0/1, Adc0_4/1, Adc0_5/1, Adc0_23/1, Adc0_22/1, Adc0_21/1, Adc0_20/1, Adc0_19/1, Adc0_18/1, Adc0_17/1, Adc0_16/1, Adc0_15/1, Adc0_14/1
  Nominal Adc Gain/1 -> Adc0_16/2, Adc0_17/2, Adc0_18/2, Adc0_19/2, Adc0_20/2, Adc0_23/2, Adc0_22/2, Adc0_21/2, Adc0_15/2, Adc0_14/2, Adc0_13/2, Adc0_12/2, Adc0_11/2, Adc0_10/2, Adc0_9/2, Adc0_8/2, Adc0_7/2, Adc0_6/2, Adc0_5/2, Adc0_4/2, Adc0_3/2, Adc0_2/2, Adc0_1/2, Adc0_0/2
  Shunt Current A/1 -> Data Type Conversion/1
  Shunt Current B/1 -> Data Type Conversion1/1
  Shunt Current C/1 -> Data Type Conversion2/1
  Data Type Conversion/1 -> Adc0_6/1, Adc0_1/1
  Data Type Conversion1/1 -> Adc0_7/1, Adc0_2/1
  Data Type Conversion2/1 -> Adc0_8/1, Adc0_3/1
  Data Type Conversion7/1 -> Adc0_13/1
  Shunt Current Reference - Inverter 1/1 -> Data Type Conversion5/1
  Data Type Conversion5/1 -> Adc0_9/1
  Data Type Conversion4/1 -> Adc0_10/1
  Data Type Conversion3/1 -> Adc0_12/1
  Data Type Conversion6/1 -> Adc0_11/1
  MotAg6Cos/1 -> Data Type Conversion7/1
  MotAg5Sin/1 -> Data Type Conversion4/1
  MotAg6Sin/1 -> Data Type Conversion3/1
  MotAg5Cos/1 -> Data Type Conversion6/1

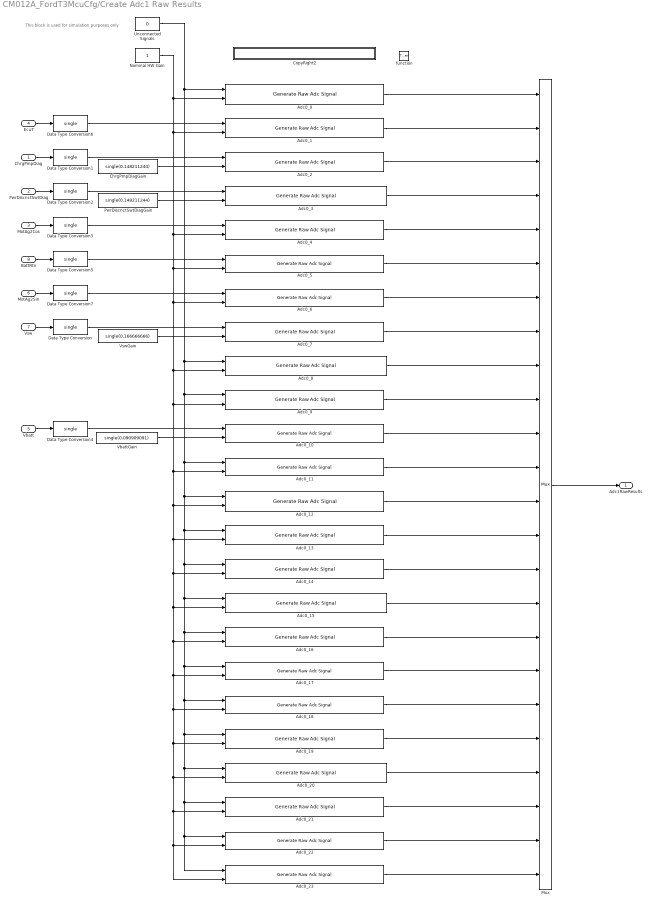
== system CM012A_FordT3McuCfg/Create Adc1 Raw Results ==
  note: This block is used for simulation purposes only
  ChrgPmpDiag : Inport  RequirementInfo={} %GIDa_e258cd79_bec5_446e_9937_0d47621c2450
  PwrDiscnctSwtDiag : Inport  RequirementInfo={} %GIDa_fd3f0e28_f46a_486f_bc1c_fda2c1e9d04a  Port=2
  MotAg2Cos : Inport  RequirementInfo={} %GIDa_782f1634_ffb7_43c0_9bac_b9f16114ad09  Port=3
  EcuT : Inport  RequirementInfo={} %GIDa_23c9caba_12da_4716_88b8_3b88f9f2ebe5  Port=4
  Vbatt : Inport  RequirementInfo={} %GIDa_345b9e4c_a7db_49fb_abbd_8077c66ef6c8  Port=5
  MotAg2Sin : Inport  RequirementInfo={} %GIDa_235a57ef_9770_4eaf_ad5b_f64c811f6eea  Port=6
  Vsw : Inport  RequirementInfo={} %GIDa_606d776e_1b77_4755_8b72_bc303eb70db1  Port=7
  BattRtn : Inport  RequirementInfo={} %GIDa_5a84aff0_8baa_4a23_848b_526bdf8c2902  Port=8
  function : TriggerPort  TriggerType=function-call
  Adc0_{0..23} (24 alike) : CM012A_FordT3McuCfg_ModelLibrary/Generate Raw Adc Signal
  ChrgPmpDiagGain : Constant  Value=single(0.148211244)  OutDataTypeStr=single
  CopyRight2 : Subsystem  Description=|  mask(Copyright Information){none=on}
      | Copyright info block.                                               
      |                                                                     
      | Place copyright information at the top of every subsystem in design.
      mask prompts: none "No parameters"
      mask help: Place copyright information at the top of every subsystem in design.
      mask Display:
      | NxtrConf = 'Nexteer Confidential';
      | 
      | sys = bdroot; %handle for the current model ("system")
      | first = get_param(sys,'Created');
      | first = first(end-3:end);  %year is last four digits
      | 
      | last = get_param(sys,'LastModifiedDate');
      | if isempty(last)
      |     last = datestr(now,'yyyy');
      | else
      |     last = last(end-3:end);
      | end
      | 
      | if strcmp(first,last)
      |     fprintf('%s -- Copyright %s Nexteer',NxtrConf,first)
      | else
      |     fprintf('%s -- %s%s- %s Nexteer',NxtrConf,char(169),first,last)
      | end
  Data Type Conversion{,1..7} (8 alike) : DataTypeConversion  OutDataTypeStr=single
  Mux : Mux  Inputs=24
  Nominal HW Gain : Constant  OutDataTypeStr=single
  PwrDiscnctSwtDiagGain : Constant  Value=single(0.148211244)  OutDataTypeStr=single
  Unconnected Signals : Constant  Value=0  OutDataTypeStr=single
  VbattGain : Constant  Value=single(0.090909091)  OutDataTypeStr=single
  VswGain : Constant  Value=single(0.166666666)  OutDataTypeStr=single
  Adc1RawResults : Outport
  wires:
  Unconnected Signals/1 -> Adc0_0/1, Adc0_8/1, Adc0_9/1, Adc0_11/1, Adc0_12/1, Adc0_13/1, Adc0_14/1, Adc0_15/1, Adc0_16/1, Adc0_17/1, Adc0_18/1, Adc0_19/1, Adc0_20/1, Adc0_21/1, Adc0_22/1, Adc0_23/1
  Adc0_23/1 -> Mux/24
  Adc0_22/1 -> Mux/23
  Adc0_21/1 -> Mux/22
  Adc0_20/1 -> Mux/21
  Adc0_19/1 -> Mux/20
  Adc0_18/1 -> Mux/19
  Adc0_17/1 -> Mux/18
  Adc0_16/1 -> Mux/17
  Adc0_15/1 -> Mux/16
  Adc0_14/1 -> Mux/15
  Adc0_13/1 -> Mux/14
  Adc0_12/1 -> Mux/13
  Adc0_11/1 -> Mux/12
  Adc0_10/1 -> Mux/11
  Adc0_9/1 -> Mux/10
  Adc0_8/1 -> Mux/9
  Adc0_7/1 -> Mux/8
  Adc0_6/1 -> Mux/7
  Adc0_5/1 -> Mux/6
  Adc0_4/1 -> Mux/5
  Adc0_3/1 -> Mux/4
  Adc0_2/1 -> Mux/3
  Adc0_1/1 -> Mux/2
  Adc0_0/1 -> Mux/1
  Mux/1 -> Adc1RawResults/1
  Nominal HW Gain/1 -> Adc0_0/2, Adc0_1/2, Adc0_4/2, Adc0_5/2, Adc0_6/2, Adc0_8/2, Adc0_9/2, Adc0_11/2, Adc0_12/2, Adc0_13/2, Adc0_14/2, Adc0_15/2, Adc0_16/2, Adc0_17/2, Adc0_18/2, Adc0_19/2, Adc0_20/2, Adc0_21/2, Adc0_22/2, Adc0_23/2
  ChrgPmpDiag/1 -> Data Type Conversion1/1
  PwrDiscnctSwtDiag/1 -> Data Type Conversion2/1
  MotAg2Cos/1 -> Data Type Conversion3/1
  Data Type Conversion1/1 -> Adc0_2/1
  Data Type Conversion2/1 -> Adc0_3/1
  Data Type Conversion3/1 -> Adc0_4/1
  Data Type Conversion5/1 -> Adc0_5/1
  EcuT/1 -> Data Type Conversion6/1
  Data Type Conversion6/1 -> Adc0_1/1
  Vbatt/1 -> Data Type Conversion4/1
  Data Type Conversion4/1 -> Adc0_10/1
  MotAg2Sin/1 -> Data Type Conversion7/1
  Data Type Conversion7/1 -> Adc0_6/1
  Vsw/1 -> Data Type Conversion/1
  Data Type Conversion/1 -> Adc0_7/1
  VswGain/1 -> Adc0_7/2
  VbattGain/1 -> Adc0_10/2
  BattRtn/1 -> Data Type Conversion5/1
  ChrgPmpDiagGain/1 -> Adc0_2/2
  PwrDiscnctSwtDiagGain/1 -> Adc0_3/2
